simulink library "Arithmetic_Operations_Lib"  (R2023a)
settings: Solver=ode45  StartTime=0.0  StopTime=10.0  RelTol=1e-3  EnableMultiTasking=on
libraries: Miscellaneous x202
(part 3 of 4)

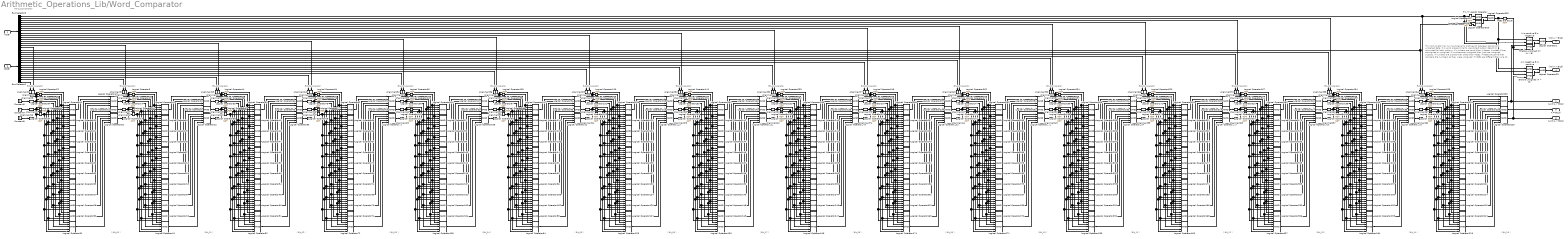
== system Arithmetic_Operations_Lib/Word_Comparator ==
  note: This comparator has no input signal to distinguish between signed and unsigned data. It is up to programmer to use correct output. Result is computed for both options.
      | If numbers are equal then it doesn`t matter if they are signed or unsigned.
      | If numbers are unsigned then just use unsigned outputs.
      | If numbers are signed then check their MSBs.
      | If MSBs are same then compare the numbers as they were unsigned.
      | If MSBs are different then one of the numbers is positive and the other one is negative. So we can immediatelly say which one is greater.
  note: Bit_Comparator
  note: ( Bit_00 )
  note: ( Bit_01 )
  note: Bit_Comparator
  note: ( Bit_02 )
  note: Bit_Comparator
  note: ( Bit_03 )
  note: Bit_Comparator
  note: ( Bit_06 )
  note: Bit_Comparator
  note: ( Bit_05 )
  note: ( Bit_04 )
  note: Bit_Comparator
  note: Bit_Comparator
  note: Bit_Comparator
  note: ( Bit_07 )
  note: Bit_Comparator
  note: Bit_Comparator
  note: ( Bit_09 )
  note: Bit_Comparator
  note: Bit_Comparator
  note: ( Bit_12 )
  note: ( Bit_13 )
  note: Bit_Comparator
  note: ( Bit_10 )
  note: ( Bit_14 )
  note: ( Bit_08 )
  note: Bit_Comparator
  note: Bit_Comparator
  note: ( Bit_11 )
  note: ( Bit_15 )
  note: Bit_Comparator
  note: Bit_Xor
  note: Word_Comparator
  A(2B) : Inport
  B(2B) : Inport  Port=2
  "A is negative B is positive " : Logic  Operator=NAND  IconShape=distinctive  AllPortsSameDT=off  OutDataTypeStr=boolean
  A is positive B is negative : Logic  Operator=NAND  IconShape=distinctive  AllPortsSameDT=off  OutDataTypeStr=boolean
  Alignment{1..75,77..81} (80 alike) : Miscellaneous/Alignment  SystemSampleTime=-1  VariantActivationTime=update diagram  Latency=0  AutoFrameSizeCalculation=off
  Bus Selector2 : BusSelector  OutputSignals=b15,b14,b13,b12,b11,b10,b09,b08,b07,b06,b05,b04,b03,b02,b01,b00
  Bus Selector3 : BusSelector  OutputSignals=b15,b14,b13,b12,b11,b10,b09,b08,b07,b06,b05,b04,b03,b02,b01,b00
  Constant3 : Constant  Value=0  OutDataTypeStr=int16
  Constant4 : Constant  OutDataTypeStr=int16
  Constant5 : Constant  Value=0  OutDataTypeStr=int16
  Enable unsigned (A < B) : Logic  Operator=NAND  IconShape=distinctive  AllPortsSameDT=off  OutDataTypeStr=boolean
  Enable unsigned (2) (A > B) : Logic  Operator=NAND  IconShape=distinctive  AllPortsSameDT=off  OutDataTypeStr=boolean
  Logical Operator{,1..2,21,29,43,63,93,95,118,140,183,208,236,238,261,283,303,317,319,326} (21 alike) : Logic  Operator=NAND  IconShape=distinctive  AllPortsSameDT=off  OutDataTypeStr=boolean
  Logical Operator{4..13,18..20,23..28,30..33,38..42,45..54,59..62,65..74,79..86,91..92,94,97..102,104..107,112..117,120..130,135..139,142..152,157..166,168..171,174,177..182,185..197,202..206,210..217,219..221,226..228,230..232,234..235,237,240..245,247..250,255..260,263..273,278..282,285..295,300..302,304..309,313,315..316,318,321,323..324} (224 alike) : Logic  Operator=NAND  Inputs=5  IconShape=distinctive  AllPortsSameDT=off  OutDataTypeStr=boolean
  Logical Operator{3,14..17,22,34..37,44,55..58,64,75..78,87..90,96,103,108..111,119,131..134,141,153..156,167,172..173,175..176,184,198..201,207,209,218,222..225,229,233,239,246,251..254,262,274..277,284,296..299,310..312,314,320,325,327} (82 alike) : Logic  Operator=NOT  IconShape=distinctive  AllPortsSameDT=off  OutDataTypeStr=boolean
  MSBs are equal : Logic  Operator=NOT  IconShape=distinctive  AllPortsSameDT=off  OutDataTypeStr=boolean
  (uint) A > B(1b) : Outport
  (uint) A < B(1b) : Outport  Port=2
  (int) A > B(1b) : Outport  Port=3
  (int) A < B(1b) : Outport  Port=4
  A = B(1b) : Outport  Port=5
  wires:
  Bus Selector3/15 -> Alignment3/1  "<b01>"
  A(2B)/1 -> Bus Selector3/1
  Bus Selector2/15 -> Alignment5/1  "<b01>"
  B(2B)/1 -> Bus Selector2/1
  "A is negative B is positive "/1 -> Logical Operator29/1
  A is positive B is negative/1 -> Logical Operator1/1
  Logical Operator29/1 -> (int) A < B(1b)/1
  Logical Operator1/1 -> (int) A > B(1b)/1
  Enable unsigned (A < B)/1 -> Logical Operator29/2
  Enable unsigned (2) (A > B)/1 -> Logical Operator1/2
  MSBs are equal/1 -> Enable unsigned (A < B)/1, Enable unsigned (2) (A > B)/2
  Logical Operator326/1 -> MSBs are equal/1, A is positive B is negative/1, "A is negative B is positive "/1
  Constant5/1 -> Alignment10/1
  Constant3/1 -> Alignment8/1
  Constant4/1 -> Alignment9/1
  Logical Operator30/1 -> Logical Operator32/4
  Logical Operator31/1 -> Logical Operator32/5
  Logical Operator33/1 -> Logical Operator32/1
  Logical Operator28/1 -> Logical Operator32/3
  Logical Operator27/1 -> Logical Operator32/2
  Logical Operator36/1 -> Logical Operator41/4, Logical Operator30/4, Logical Operator31/4, Logical Operator27/4, Logical Operator33/4, Logical Operator26/4, Logical Operator25/4, Logical Operator23/4
  Logical Operator37/1 -> Logical Operator41/5, Logical Operator28/5, Logical Operator30/5, Logical Operator39/5, Logical Operator38/5, Logical Operator26/5, Logical Operator25/5, Logical Operator24/5
  Logical Operator34/1 -> Logical Operator41/2, Logical Operator39/2, Logical Operator33/2, Logical Operator25/2, Logical Operator24/2, Logical Operator23/2
  Logical Operator22/1 -> Logical Operator41/1, Logical Operator30/1, Logical Operator28/1, Logical Operator27/1, Logical Operator33/1, Logical Operator39/1
  Logical Operator35/1 -> Logical Operator28/3, Logical Operator31/3, Logical Operator27/3, Logical Operator33/3, Logical Operator39/3, Logical Operator38/3, Logical Operator24/3, Logical Operator23/3
  Logical Operator38/1 -> Logical Operator21/1
  Logical Operator39/1 -> Logical Operator21/2
  Logical Operator26/1 -> Logical Operator40/5
  Logical Operator24/1 -> Logical Operator40/3
  Logical Operator23/1 -> Logical Operator40/2
  Logical Operator25/1 -> Logical Operator40/4
  Logical Operator41/1 -> Logical Operator40/1
  Alignment1/1 -> Logical Operator31/1, Logical Operator38/1, Logical Operator26/1, Logical Operator25/1, Logical Operator24/1, Logical Operator23/1, Logical Operator22/1
  Alignment2/1 -> Logical Operator30/2, Logical Operator31/2, Logical Operator28/2, Logical Operator27/2, Logical Operator38/2, Logical Operator26/2, Logical Operator34/1
  Alignment8/1 -> Logical Operator41/3, Logical Operator26/3, Logical Operator30/3, Logical Operator25/3, Logical Operator35/1
  Alignment9/1 -> Logical Operator36/1, Logical Operator28/4, Logical Operator39/4, Logical Operator38/4, Logical Operator24/4
  Alignment10/1 -> Logical Operator37/1, Logical Operator27/5, Logical Operator31/5, Logical Operator33/5, Logical Operator23/5
  Logical Operator42/1 -> Logical Operator20/1
  Logical Operator6/1 -> Logical Operator20/4
  Alignment3/1 -> Logical Operator11/1, Logical Operator18/1, Logical Operator7/1, Logical Operator6/1, Logical Operator5/1, Logical Operator4/1, Logical Operator3/1
  Logical Operator14/1 -> Logical Operator42/2, Logical Operator19/2, Logical Operator13/2, Logical Operator6/2, Logical Operator5/2, Logical Operator4/2
  Logical Operator3/1 -> Logical Operator42/1, Logical Operator10/1, Logical Operator9/1, Logical Operator8/1, Logical Operator13/1, Logical Operator19/1
  Logical Operator17/1 -> Logical Operator42/5, Logical Operator9/5, Logical Operator10/5, Logical Operator19/5, Logical Operator18/5, Logical Operator7/5, Logical Operator6/5, Logical Operator5/5
  Logical Operator15/1 -> Logical Operator9/3, Logical Operator11/3, Logical Operator8/3, Logical Operator13/3, Logical Operator19/3, Logical Operator18/3, Logical Operator5/3, Logical Operator4/3
  Logical Operator16/1 -> Logical Operator42/4, Logical Operator10/4, Logical Operator11/4, Logical Operator8/4, Logical Operator13/4, Logical Operator7/4, Logical Operator6/4, Logical Operator4/4
  Logical Operator9/1 -> Logical Operator12/3
  Logical Operator10/1 -> Logical Operator12/4
  Logical Operator18/1 -> Logical Operator2/1
  Logical Operator7/1 -> Logical Operator20/5
  Logical Operator13/1 -> Logical Operator12/1
  Alignment7/1 -> Logical Operator16/1, Logical Operator9/4, Logical Operator19/4, Logical Operator18/4, Logical Operator5/4
  Logical Operator11/1 -> Logical Operator12/5
  Alignment4/1 -> Logical Operator17/1, Logical Operator8/5, Logical Operator11/5, Logical Operator13/5, Logical Operator4/5
  Alignment5/1 -> Logical Operator10/2, Logical Operator11/2, Logical Operator9/2, Logical Operator8/2, Logical Operator18/2, Logical Operator7/2, Logical Operator14/1
  Logical Operator19/1 -> Logical Operator2/2
  Alignment6/1 -> Logical Operator42/3, Logical Operator7/3, Logical Operator10/3, Logical Operator6/3, Logical Operator15/1
  Logical Operator8/1 -> Logical Operator12/2
  Logical Operator5/1 -> Logical Operator20/3
  Logical Operator4/1 -> Logical Operator20/2
  Logical Operator62/1 -> Logical Operator61/1
  Logical Operator47/1 -> Logical Operator61/4
  Alignment11/1 -> Logical Operator52/1, Logical Operator59/1, Logical Operator48/1, Logical Operator47/1, Logical Operator46/1, Logical Operator45/1, Logical Operator44/1
  Logical Operator55/1 -> Logical Operator62/2, Logical Operator60/2, Logical Operator54/2, Logical Operator47/2, Logical Operator46/2, Logical Operator45/2
  Logical Operator44/1 -> Logical Operator62/1, Logical Operator51/1, Logical Operator50/1, Logical Operator49/1, Logical Operator54/1, Logical Operator60/1
  Logical Operator58/1 -> Logical Operator62/5, Logical Operator50/5, Logical Operator51/5, Logical Operator60/5, Logical Operator59/5, Logical Operator48/5, Logical Operator47/5, Logical Operator46/5
  Logical Operator56/1 -> Logical Operator50/3, Logical Operator52/3, Logical Operator49/3, Logical Operator54/3, Logical Operator60/3, Logical Operator59/3, Logical Operator46/3, Logical Operator45/3
  Logical Operator57/1 -> Logical Operator62/4, Logical Operator51/4, Logical Operator52/4, Logical Operator49/4, Logical Operator54/4, Logical Operator48/4, Logical Operator47/4, Logical Operator45/4
  Logical Operator50/1 -> Logical Operator53/3
  Logical Operator51/1 -> Logical Operator53/4
  Logical Operator59/1 -> Logical Operator43/1
  Logical Operator48/1 -> Logical Operator61/5
  Logical Operator54/1 -> Logical Operator53/1
  Alignment15/1 -> Logical Operator57/1, Logical Operator50/4, Logical Operator60/4, Logical Operator59/4, Logical Operator46/4
  Logical Operator52/1 -> Logical Operator53/5
  Alignment12/1 -> Logical Operator58/1, Logical Operator49/5, Logical Operator52/5, Logical Operator54/5, Logical Operator45/5
  Alignment13/1 -> Logical Operator51/2, Logical Operator52/2, Logical Operator50/2, Logical Operator49/2, Logical Operator59/2, Logical Operator48/2, Logical Operator55/1
  Logical Operator60/1 -> Logical Operator43/2
  Alignment14/1 -> Logical Operator62/3, Logical Operator48/3, Logical Operator51/3, Logical Operator47/3, Logical Operator56/1
  Logical Operator49/1 -> Logical Operator53/2
  Logical Operator46/1 -> Logical Operator61/3
  Logical Operator45/1 -> Logical Operator61/2
  Logical Operator82/1 -> Logical Operator81/1
  Logical Operator67/1 -> Logical Operator81/4
  Alignment16/1 -> Logical Operator72/1, Logical Operator79/1, Logical Operator68/1, Logical Operator67/1, Logical Operator66/1, Logical Operator65/1, Logical Operator64/1
  Logical Operator75/1 -> Logical Operator82/2, Logical Operator80/2, Logical Operator74/2, Logical Operator67/2, Logical Operator66/2, Logical Operator65/2
  Logical Operator64/1 -> Logical Operator82/1, Logical Operator71/1, Logical Operator70/1, Logical Operator69/1, Logical Operator74/1, Logical Operator80/1
  Logical Operator78/1 -> Logical Operator82/5, Logical Operator70/5, Logical Operator71/5, Logical Operator80/5, Logical Operator79/5, Logical Operator68/5, Logical Operator67/5, Logical Operator66/5
  Logical Operator76/1 -> Logical Operator70/3, Logical Operator72/3, Logical Operator69/3, Logical Operator74/3, Logical Operator80/3, Logical Operator79/3, Logical Operator66/3, Logical Operator65/3
  Logical Operator77/1 -> Logical Operator82/4, Logical Operator71/4, Logical Operator72/4, Logical Operator69/4, Logical Operator74/4, Logical Operator68/4, Logical Operator67/4, Logical Operator65/4
  Logical Operator70/1 -> Logical Operator73/3
  Logical Operator71/1 -> Logical Operator73/4
  Logical Operator79/1 -> Logical Operator63/1
  Logical Operator68/1 -> Logical Operator81/5
  Logical Operator74/1 -> Logical Operator73/1
  Alignment20/1 -> Logical Operator77/1, Logical Operator70/4, Logical Operator80/4, Logical Operator79/4, Logical Operator66/4
  Logical Operator72/1 -> Logical Operator73/5
  Alignment17/1 -> Logical Operator78/1, Logical Operator69/5, Logical Operator72/5, Logical Operator74/5, Logical Operator65/5
  Alignment18/1 -> Logical Operator71/2, Logical Operator72/2, Logical Operator70/2, Logical Operator69/2, Logical Operator79/2, Logical Operator68/2, Logical Operator75/1
  Logical Operator80/1 -> Logical Operator63/2
  Alignment19/1 -> Logical Operator82/3, Logical Operator68/3, Logical Operator71/3, Logical Operator67/3, Logical Operator76/1
  Logical Operator69/1 -> Logical Operator73/2
  Logical Operator66/1 -> Logical Operator81/3
  Logical Operator65/1 -> Logical Operator81/2
  Logical Operator61/1 -> Alignment19/1
  Logical Operator43/1 -> Alignment20/1
  Logical Operator53/1 -> Alignment17/1
  Logical Operator20/1 -> Alignment14/1
  Logical Operator2/1 -> Alignment15/1
  Logical Operator12/1 -> Alignment12/1
  Logical Operator40/1 -> Alignment6/1
  Logical Operator21/1 -> Alignment7/1
  Logical Operator32/1 -> Alignment4/1
  Logical Operator145/1 -> Logical Operator160/5
  Logical Operator157/1 -> Logical Operator140/1
  Logical Operator152/1 -> Logical Operator151/1
  Logical Operator149/1 -> Logical Operator151/4
  Logical Operator154/1 -> Logical Operator148/3, Logical Operator150/3, Logical Operator146/3, Logical Operator152/3, Logical Operator159/3, Logical Operator157/3, Logical Operator143/3, Logical Operator142/3
  Logical Operator155/1 -> Logical Operator161/4, Logical Operator149/4, Logical Operator150/4, Logical Operator146/4, Logical Operator152/4, Logical Operator145/4, Logical Operator144/4, Logical Operator142/4
  Logical Operator148/1 -> Logical Operator151/3
  Alignment28/1 -> Logical Operator150/1, Logical Operator157/1, Logical Operator145/1, Logical Operator144/1, Logical Operator143/1, Logical Operator142/1, Logical Operator141/1
  Logical Operator144/1 -> Logical Operator160/4
  Logical Operator118/1 -> Alignment33/1
  Logical Operator106/1 -> Alignment35/1
  Logical Operator117/1 -> Logical Operator94/1
  Logical Operator161/1 -> Logical Operator160/1
  Logical Operator129/1 -> Alignment29/1
  Logical Operator124/1 -> Logical Operator129/2
  Alignment26/1 -> Logical Operator139/3, Logical Operator123/3, Logical Operator127/3, Logical Operator122/3, Logical Operator132/1
  Alignment25/1 -> Logical Operator127/2, Logical Operator128/2, Logical Operator126/2, Logical Operator124/2, Logical Operator135/2, Logical Operator123/2, Logical Operator131/1
  Logical Operator137/1 -> Logical Operator118/2
  Alignment27/1 -> Logical Operator133/1, Logical Operator126/4, Logical Operator137/4, Logical Operator135/4, Logical Operator121/4
  Alignment24/1 -> Logical Operator134/1, Logical Operator124/5, Logical Operator128/5, Logical Operator130/5, Logical Operator120/5
  Logical Operator128/1 -> Logical Operator129/5
  Alignment33/1 -> Logical Operator155/1, Logical Operator148/4, Logical Operator159/4, Logical Operator157/4, Logical Operator143/4
  Logical Operator130/1 -> Logical Operator129/1
  Logical Operator141/1 -> Logical Operator161/1, Logical Operator149/1, Logical Operator148/1, Logical Operator146/1, Logical Operator152/1, Logical Operator159/1
  Logical Operator119/1 -> Logical Operator139/1, Logical Operator127/1, Logical Operator126/1, Logical Operator124/1, Logical Operator130/1, Logical Operator137/1
  Alignment23/1 -> Logical Operator128/1, Logical Operator135/1, Logical Operator123/1, Logical Operator122/1, Logical Operator121/1, Logical Operator120/1, Logical Operator119/1
  Logical Operator131/1 -> Logical Operator139/2, Logical Operator137/2, Logical Operator130/2, Logical Operator122/2, Logical Operator121/2, Logical Operator120/2
  Alignment29/1 -> Logical Operator156/1, Logical Operator146/5, Logical Operator150/5, Logical Operator152/5, Logical Operator142/5
  Logical Operator156/1 -> Logical Operator161/5, Logical Operator148/5, Logical Operator149/5, Logical Operator159/5, Logical Operator157/5, Logical Operator145/5, Logical Operator144/5, Logical Operator143/5
  Logical Operator138/1 -> Alignment31/1
  Logical Operator123/1 -> Logical Operator138/5
  Alignment36/1 -> Logical Operator83/2, Logical Operator84/2, Logical Operator162/2, Logical Operator158/2, Logical Operator91/2, Logical Operator147/2, Logical Operator87/1
  Logical Operator93/1 -> Alignment27/1
  Alignment35/1 -> Logical Operator90/1, Logical Operator158/5, Logical Operator84/5, Logical Operator86/5, Logical Operator114/5
  Alignment38/1 -> Logical Operator89/1, Logical Operator162/4, Logical Operator92/4, Logical Operator91/4, Logical Operator125/4
  Logical Operator95/1 -> Alignment38/1
  Logical Operator94/1 -> Alignment26/1
  Logical Operator99/1 -> Logical Operator115/4
  Logical Operator121/1 -> Logical Operator138/3
  Alignment21/1 -> Logical Operator105/1, Logical Operator112/1, Logical Operator100/1, Logical Operator99/1, Logical Operator98/1, Logical Operator97/1, Logical Operator96/1
  Logical Operator136/1 -> Logical Operator94/4
  Logical Operator108/1 -> Logical Operator116/2, Logical Operator113/2, Logical Operator107/2, Logical Operator99/2, Logical Operator98/2, Logical Operator97/2
  Logical Operator84/1 -> Logical Operator85/5
  Logical Operator96/1 -> Logical Operator116/1, Logical Operator104/1, Logical Operator102/1, Logical Operator101/1, Logical Operator107/1, Logical Operator113/1
  Logical Operator111/1 -> Logical Operator116/5, Logical Operator102/5, Logical Operator104/5, Logical Operator113/5, Logical Operator112/5, Logical Operator100/5, Logical Operator99/5, Logical Operator98/5
  Logical Operator126/1 -> Logical Operator129/3
  Logical Operator110/1 -> Logical Operator116/4, Logical Operator104/4, Logical Operator105/4, Logical Operator101/4, Logical Operator107/4, Logical Operator100/4, Logical Operator99/4, Logical Operator97/4
  Logical Operator107/1 -> Logical Operator106/1
  Logical Operator102/1 -> Logical Operator106/3
  Logical Operator105/1 -> Logical Operator106/5
  Logical Operator113/1 -> Logical Operator95/2
  Logical Operator100/1 -> Logical Operator115/5
  Logical Operator142/1 -> Logical Operator160/2
  Logical Operator135/1 -> Logical Operator118/1
  Logical Operator127/1 -> Logical Operator129/4
  Logical Operator109/1 -> Logical Operator102/3, Logical Operator105/3, Logical Operator101/3, Logical Operator107/3, Logical Operator113/3, Logical Operator112/3, Logical Operator98/3, Logical Operator97/3
  Logical Operator133/1 -> Logical Operator139/4, Logical Operator127/4, Logical Operator128/4, Logical Operator124/4, Logical Operator130/4, Logical Operator123/4, Logical Operator122/4, Logical Operator120/4
  Logical Operator92/1 -> Logical Operator93/2
  Logical Operator116/1 -> Logical Operator115/1
  Logical Operator90/1 -> Logical Operator117/5, Logical Operator162/5, Logical Operator83/5, Logical Operator92/5, Logical Operator91/5, Logical Operator147/5, Logical Operator136/5, Logical Operator125/5
  Logical Operator85/1 -> Alignment24/1
  Logical Operator104/1 -> Logical Operator106/4
  Logical Operator132/1 -> Logical Operator126/3, Logical Operator128/3, Logical Operator124/3, Logical Operator130/3, Logical Operator137/3, Logical Operator135/3, Logical Operator121/3, Logical Operator120/3
  Logical Operator115/1 -> Alignment37/1
  Logical Operator146/1 -> Logical Operator151/2
  Alignment31/1 -> Logical Operator161/3, Logical Operator145/3, Logical Operator149/3, Logical Operator144/3, Logical Operator154/1
  Logical Operator150/1 -> Logical Operator151/5
  Logical Operator112/1 -> Logical Operator95/1
  Logical Operator139/1 -> Logical Operator138/1
  Alignment30/1 -> Logical Operator149/2, Logical Operator150/2, Logical Operator148/2, Logical Operator146/2, Logical Operator157/2, Logical Operator145/2, Logical Operator153/1
  Logical Operator158/1 -> Logical Operator85/2
  Logical Operator86/1 -> Logical Operator85/1
  Logical Operator147/1 -> Logical Operator94/5
  Logical Operator162/1 -> Logical Operator85/3
  Logical Operator87/1 -> Logical Operator117/2, Logical Operator92/2, Logical Operator86/2, Logical Operator136/2, Logical Operator125/2, Logical Operator114/2
  Logical Operator114/1 -> Logical Operator94/2
  Logical Operator83/1 -> Logical Operator85/4
  Logical Operator91/1 -> Logical Operator93/1
  Alignment37/1 -> Logical Operator117/3, Logical Operator147/3, Logical Operator83/3, Logical Operator136/3, Logical Operator88/1
  Logical Operator159/1 -> Logical Operator140/2
  Logical Operator143/1 -> Logical Operator160/3
  Logical Operator88/1 -> Logical Operator162/3, Logical Operator84/3, Logical Operator158/3, Logical Operator86/3, Logical Operator92/3, Logical Operator91/3, Logical Operator125/3, Logical Operator114/3
  Alignment34/1 -> Logical Operator84/1, Logical Operator91/1, Logical Operator147/1, Logical Operator136/1, Logical Operator125/1, Logical Operator114/1, Logical Operator103/1
  Alignment40/1 -> Logical Operator110/1, Logical Operator102/4, Logical Operator113/4, Logical Operator112/4, Logical Operator98/4
  Alignment22/1 -> Logical Operator111/1, Logical Operator101/5, Logical Operator105/5, Logical Operator107/5, Logical Operator97/5
  Logical Operator89/1 -> Logical Operator117/4, Logical Operator83/4, Logical Operator84/4, Logical Operator158/4, Logical Operator86/4, Logical Operator147/4, Logical Operator136/4, Logical Operator114/4
  Logical Operator120/1 -> Logical Operator138/2
  Alignment32/1 -> Logical Operator104/2, Logical Operator105/2, Logical Operator102/2, Logical Operator101/2, Logical Operator112/2, Logical Operator100/2, Logical Operator108/1
  Logical Operator103/1 -> Logical Operator117/1, Logical Operator83/1, Logical Operator162/1, Logical Operator158/1, Logical Operator86/1, Logical Operator92/1
  Logical Operator153/1 -> Logical Operator161/2, Logical Operator159/2, Logical Operator152/2, Logical Operator144/2, Logical Operator143/2, Logical Operator142/2
  Alignment39/1 -> Logical Operator116/3, Logical Operator100/3, Logical Operator104/3, Logical Operator99/3, Logical Operator109/1
  Logical Operator101/1 -> Logical Operator106/2
  Logical Operator134/1 -> Logical Operator139/5, Logical Operator126/5, Logical Operator127/5, Logical Operator137/5, Logical Operator135/5, Logical Operator123/5, Logical Operator122/5, Logical Operator121/5
  Logical Operator98/1 -> Logical Operator115/3
  Logical Operator97/1 -> Logical Operator115/2
  Logical Operator122/1 -> Logical Operator138/4
  Logical Operator125/1 -> Logical Operator94/3
  Logical Operator288/1 -> Logical Operator304/5
  Logical Operator300/1 -> Logical Operator283/1
  Logical Operator295/1 -> Logical Operator294/1
  Logical Operator292/1 -> Logical Operator294/4
  Logical Operator297/1 -> Logical Operator291/3, Logical Operator293/3, Logical Operator289/3, Logical Operator295/3, Logical Operator302/3, Logical Operator300/3, Logical Operator286/3, Logical Operator285/3
  Logical Operator298/1 -> Logical Operator305/4, Logical Operator292/4, Logical Operator293/4, Logical Operator289/4, Logical Operator295/4, Logical Operator288/4, Logical Operator287/4, Logical Operator285/4
  Logical Operator291/1 -> Logical Operator294/3
  Alignment53/1 -> Logical Operator298/1, Logical Operator291/4, Logical Operator302/4, Logical Operator300/4, Logical Operator286/4
  Logical Operator299/1 -> Logical Operator305/5, Logical Operator291/5, Logical Operator292/5, Logical Operator302/5, Logical Operator300/5, Logical Operator288/5, Logical Operator287/5, Logical Operator286/5
  Logical Operator287/1 -> Logical Operator304/4
  Logical Operator305/1 -> Logical Operator304/1
  Logical Operator236/1 -> Alignment47/1
  Logical Operator238/1 -> Alignment79/1
  Logical Operator249/1 -> Alignment74/1
  Logical Operator272/1 -> Alignment49/1
  Logical Operator264/1 -> Logical Operator281/3
  Logical Operator267/1 -> Logical Operator272/2
  Alignment46/1 -> Logical Operator282/3, Logical Operator266/3, Logical Operator270/3, Logical Operator265/3, Logical Operator275/1
  Alignment45/1 -> Logical Operator270/2, Logical Operator271/2, Logical Operator269/2, Logical Operator267/2, Logical Operator278/2, Logical Operator266/2, Logical Operator274/1
  Alignment47/1 -> Logical Operator276/1, Logical Operator269/4, Logical Operator280/4, Logical Operator278/4, Logical Operator264/4
  Logical Operator271/1 -> Logical Operator272/5
  Logical Operator266/1 -> Logical Operator281/5
  Logical Operator296/1 -> Logical Operator305/2, Logical Operator302/2, Logical Operator295/2, Logical Operator287/2, Logical Operator286/2, Logical Operator285/2
  Logical Operator277/1 -> Logical Operator282/5, Logical Operator269/5, Logical Operator270/5, Logical Operator280/5, Logical Operator278/5, Logical Operator266/5, Logical Operator265/5, Logical Operator264/5
  Logical Operator262/1 -> Logical Operator282/1, Logical Operator270/1, Logical Operator269/1, Logical Operator267/1, Logical Operator273/1, Logical Operator280/1
  Alignment43/1 -> Logical Operator271/1, Logical Operator278/1, Logical Operator266/1, Logical Operator265/1, Logical Operator264/1, Logical Operator263/1, Logical Operator262/1
  Alignment49/1 -> Logical Operator299/1, Logical Operator289/5, Logical Operator293/5, Logical Operator295/5, Logical Operator285/5
  Logical Operator281/1 -> Alignment51/1
  Logical Operator197/1 -> Logical Operator195/1
  Alignment57/1 -> Logical Operator201/1, Logical Operator190/5, Logical Operator194/5, Logical Operator197/5, Logical Operator186/5
  Logical Operator189/1 -> Logical Operator205/5
  Logical Operator194/1 -> Logical Operator195/5
  Logical Operator204/1 -> Logical Operator183/2
  Alignment58/1 -> Logical Operator193/2, Logical Operator194/2, Logical Operator192/2, Logical Operator190/2, Logical Operator202/2, Logical Operator189/2, Logical Operator198/1
  Logical Operator190/1 -> Logical Operator195/2
  Logical Operator170/1 -> Alignment69/1
  Logical Operator182/1 -> Logical Operator318/1
  Logical Operator284/1 -> Logical Operator305/1, Logical Operator292/1, Logical Operator291/1, Logical Operator289/1, Logical Operator295/1, Logical Operator302/1
  Logical Operator260/1 -> Logical Operator237/1
  Logical Operator184/1 -> Logical Operator206/1, Logical Operator193/1, Logical Operator192/1, Logical Operator190/1, Logical Operator197/1, Logical Operator204/1
  Logical Operator166/1 -> Logical Operator170/3
  Logical Operator175/1 -> Logical Operator181/4, Logical Operator168/4, Logical Operator169/4, Logical Operator165/4, Logical Operator171/4, Logical Operator164/4, Logical Operator324/4, Logical Operator321/4
  Logical Operator192/1 -> Logical Operator195/3
  Alignment44/1 -> Logical Operator277/1, Logical Operator267/5, Logical Operator271/5, Logical Operator273/5, Logical Operator263/5
  Logical Operator307/1 -> Logical Operator308/5
  Alignment48/1 -> Logical Operator293/1, Logical Operator300/1, Logical Operator288/1, Logical Operator287/1, Logical Operator286/1, Logical Operator285/1, Logical Operator284/1
  Logical Operator172/1 -> Logical Operator181/2, Logical Operator178/2, Logical Operator171/2, Logical Operator324/2, Logical Operator323/2, Logical Operator321/2
  Logical Operator203/1 -> Logical Operator318/4
  Alignment54/1 -> Logical Operator169/1, Logical Operator177/1, Logical Operator164/1, Logical Operator324/1, Logical Operator323/1, Logical Operator321/1, Logical Operator320/1
  Logical Operator169/1 -> Logical Operator170/5
  Logical Operator178/1 -> Logical Operator319/2
  Logical Operator200/1 -> Logical Operator206/4, Logical Operator193/4, Logical Operator194/4, Logical Operator190/4, Logical Operator197/4, Logical Operator189/4, Logical Operator188/4, Logical Operator186/4
  Logical Operator186/1 -> Logical Operator205/2
  Logical Operator312/1 -> Logical Operator182/4, Logical Operator306/4, Logical Operator307/4, Logical Operator227/4, Logical Operator309/4, Logical Operator215/4, Logical Operator203/4, Logical Operator179/4
  Alignment75/1 -> Logical Operator175/1, Logical Operator166/4, Logical Operator178/4, Logical Operator177/4, Logical Operator323/4
  Logical Operator273/1 -> Logical Operator272/1
  Alignment55/1 -> Logical Operator176/1, Logical Operator165/5, Logical Operator169/5, Logical Operator171/5, Logical Operator321/5
  Alignment68/1 -> Logical Operator307/1, Logical Operator315/1, Logical Operator215/1, Logical Operator203/1, Logical Operator191/1, Logical Operator179/1, Logical Operator167/1
  Logical Operator280/1 -> Logical Operator261/2
  Logical Operator232/1 -> Logical Operator308/3
  Logical Operator193/1 -> Logical Operator195/4
  Logical Operator177/1 -> Logical Operator319/1
  Logical Operator215/1 -> Logical Operator318/5
  Logical Operator199/1 -> Logical Operator192/3, Logical Operator194/3, Logical Operator190/3, Logical Operator197/3, Logical Operator204/3, Logical Operator202/3, Logical Operator187/3, Logical Operator186/3
  Logical Operator310/1 -> Logical Operator182/2, Logical Operator316/2, Logical Operator309/2, Logical Operator203/2, Logical Operator191/2, Logical Operator179/2
  Logical Operator314/1 -> Logical Operator182/5, Logical Operator232/5, Logical Operator306/5, Logical Operator316/5, Logical Operator315/5, Logical Operator215/5, Logical Operator203/5, Logical Operator191/5
  Logical Operator308/1 -> Alignment57/1
  Logical Operator181/1 -> Logical Operator180/1
  Logical Operator165/1 -> Logical Operator170/2
  Logical Operator315/1 -> Logical Operator317/1
  Logical Operator311/1 -> Logical Operator232/3, Logical Operator307/3, Logical Operator227/3, Logical Operator309/3, Logical Operator316/3, Logical Operator315/3, Logical Operator191/3, Logical Operator179/3
  Logical Operator164/1 -> Logical Operator180/5
  Alignment74/1 -> Logical Operator233/1, Logical Operator301/5, Logical Operator174/5, Logical Operator196/5, Logical Operator257/5
  Alignment79/1 -> Logical Operator229/1, Logical Operator313/4, Logical Operator235/4, Logical Operator234/4, Logical Operator268/4
  Logical Operator316/1 -> Logical Operator317/2
  Logical Operator167/1 -> Logical Operator182/1, Logical Operator306/1, Logical Operator232/1, Logical Operator227/1, Logical Operator309/1, Logical Operator316/1
  Logical Operator274/1 -> Logical Operator282/2, Logical Operator280/2, Logical Operator273/2, Logical Operator265/2, Logical Operator264/2, Logical Operator263/2
  Logical Operator198/1 -> Logical Operator206/2, Logical Operator204/2, Logical Operator197/2, Logical Operator188/2, Logical Operator187/2, Logical Operator186/2
  Logical Operator237/1 -> Alignment46/1
  Logical Operator242/1 -> Logical Operator258/4
  Alignment41/1 -> Logical Operator248/1, Logical Operator255/1, Logical Operator243/1, Logical Operator242/1, Logical Operator241/1, Logical Operator240/1, Logical Operator239/1
  Alignment60/1 -> Logical Operator200/1, Logical Operator192/4, Logical Operator204/4, Logical Operator202/4, Logical Operator187/4
  Logical Operator251/1 -> Logical Operator259/2, Logical Operator256/2, Logical Operator250/2, Logical Operator242/2, Logical Operator241/2, Logical Operator240/2
  Logical Operator168/1 -> Logical Operator170/4
  Logical Operator174/1 -> Logical Operator185/5
  Logical Operator239/1 -> Logical Operator259/1, Logical Operator247/1, Logical Operator245/1, Logical Operator244/1, Logical Operator250/1, Logical Operator256/1
  Logical Operator254/1 -> Logical Operator259/5, Logical Operator245/5, Logical Operator247/5, Logical Operator256/5, Logical Operator255/5, Logical Operator243/5, Logical Operator242/5, Logical Operator241/5
  Logical Operator261/1 -> Alignment53/1
  Alignment69/1 -> Logical Operator314/1, Logical Operator227/5, Logical Operator307/5, Logical Operator309/5, Logical Operator179/5
  Logical Operator320/1 -> Logical Operator181/1, Logical Operator168/1, Logical Operator166/1, Logical Operator165/1, Logical Operator171/1, Logical Operator178/1
  Logical Operator306/1 -> Logical Operator308/4
  Logical Operator269/1 -> Logical Operator272/3
  Alignment71/1 -> Logical Operator182/3, Logical Operator215/3, Logical Operator306/3, Logical Operator203/3, Logical Operator311/1
  Logical Operator250/1 -> Logical Operator249/1
  Logical Operator309/1 -> Logical Operator308/1
  Logical Operator245/1 -> Logical Operator249/3
  Logical Operator248/1 -> Logical Operator249/5
  Alignment73/1 -> Logical Operator181/3, Logical Operator164/3, Logical Operator168/3, Logical Operator324/3, Logical Operator173/1
  Logical Operator256/1 -> Logical Operator238/2
  Logical Operator243/1 -> Logical Operator258/5
  Logical Operator285/1 -> Logical Operator304/2
  Alignment56/1 -> Logical Operator194/1, Logical Operator202/1, Logical Operator189/1, Logical Operator188/1, Logical Operator187/1, Logical Operator186/1, Logical Operator184/1
  Logical Operator278/1 -> Logical Operator261/1
  Logical Operator270/1 -> Logical Operator272/4
  Logical Operator252/1 -> Logical Operator245/3, Logical Operator248/3, Logical Operator244/3, Logical Operator250/3, Logical Operator256/3, Logical Operator255/3, Logical Operator241/3, Logical Operator240/3
  Logical Operator235/1 -> Logical Operator236/2
  Logical Operator202/1 -> Logical Operator183/1
  Logical Operator259/1 -> Logical Operator258/1
  Logical Operator233/1 -> Logical Operator260/5, Logical Operator313/5, Logical Operator163/5, Logical Operator235/5, Logical Operator234/5, Logical Operator290/5, Logical Operator279/5, Logical Operator268/5
  Logical Operator185/1 -> Alignment44/1
  Logical Operator247/1 -> Logical Operator249/4
  Logical Operator275/1 -> Logical Operator269/3, Logical Operator271/3, Logical Operator267/3, Logical Operator273/3, Logical Operator280/3, Logical Operator278/3, Logical Operator264/3, Logical Operator263/3
  Logical Operator227/1 -> Logical Operator308/2
  Logical Operator318/1 -> Alignment59/1
  Logical Operator258/1 -> Alignment78/1
  Alignment51/1 -> Logical Operator305/3, Logical Operator288/3, Logical Operator292/3, Logical Operator287/3, Logical Operator297/1
  Logical Operator324/1 -> Logical Operator180/4
  Logical Operator179/1 -> Logical Operator318/2
  Logical Operator293/1 -> Logical Operator294/5
  Logical Operator282/1 -> Logical Operator281/1
  Alignment50/1 -> Logical Operator292/2, Logical Operator293/2, Logical Operator291/2, Logical Operator289/2, Logical Operator300/2, Logical Operator288/2, Logical Operator296/1
  Alignment78/1 -> Logical Operator260/3, Logical Operator290/3, Logical Operator163/3, Logical Operator279/3, Logical Operator218/1
  Logical Operator301/1 -> Logical Operator185/2
  Logical Operator171/1 -> Logical Operator170/1
  Logical Operator218/1 -> Logical Operator313/3, Logical Operator174/3, Logical Operator301/3, Logical Operator196/3, Logical Operator235/3, Logical Operator234/3, Logical Operator268/3, Logical Operator257/3
  Logical Operator286/1 -> Logical Operator304/3
  Logical Operator196/1 -> Logical Operator185/1
  Logical Operator290/1 -> Logical Operator237/5
  Logical Operator234/1 -> Logical Operator236/1
  Logical Operator163/1 -> Logical Operator185/4
  Logical Operator313/1 -> Logical Operator185/3
  Logical Operator207/1 -> Logical Operator260/2, Logical Operator235/2, Logical Operator196/2, Logical Operator279/2, Logical Operator268/2, Logical Operator257/2
  Logical Operator229/1 -> Logical Operator260/4, Logical Operator163/4, Logical Operator174/4, Logical Operator301/4, Logical Operator196/4, Logical Operator290/4, Logical Operator279/4, Logical Operator257/4
  Logical Operator206/1 -> Logical Operator205/1
  Logical Operator191/1 -> Logical Operator318/3
  Logical Operator188/1 -> Logical Operator205/4
  Logical Operator289/1 -> Logical Operator294/2
  Logical Operator201/1 -> Logical Operator206/5, Logical Operator192/5, Logical Operator193/5, Logical Operator204/5, Logical Operator202/5, Logical Operator189/5, Logical Operator188/5, Logical Operator187/5
  Alignment77/1 -> Logical Operator163/2, Logical Operator174/2, Logical Operator313/2, Logical Operator301/2, Logical Operator234/2, Logical Operator290/2, Logical Operator207/1
  Logical Operator321/1 -> Logical Operator180/2
  Logical Operator323/1 -> Logical Operator180/3
  Logical Operator319/1 -> Alignment72/1
  Alignment42/1 -> Logical Operator254/1, Logical Operator244/5, Logical Operator248/5, Logical Operator250/5, Logical Operator240/5
  Logical Operator302/1 -> Logical Operator283/2
  Alignment63/1 -> Logical Operator174/1, Logical Operator234/1, Logical Operator290/1, Logical Operator279/1, Logical Operator268/1, Logical Operator257/1, Logical Operator246/1
  Alignment81/1 -> Logical Operator253/1, Logical Operator245/4, Logical Operator256/4, Logical Operator255/4, Logical Operator241/4
  Alignment80/1 -> Logical Operator259/3, Logical Operator243/3, Logical Operator247/3, Logical Operator242/3, Logical Operator252/1
  Alignment66/1 -> Logical Operator168/2, Logical Operator169/2, Logical Operator166/2, Logical Operator165/2, Logical Operator177/2, Logical Operator164/2, Logical Operator172/1
  Logical Operator246/1 -> Logical Operator260/1, Logical Operator163/1, Logical Operator313/1, Logical Operator301/1, Logical Operator196/1, Logical Operator235/1
  Logical Operator276/1 -> Logical Operator282/4, Logical Operator270/4, Logical Operator271/4, Logical Operator267/4, Logical Operator273/4, Logical Operator266/4, Logical Operator265/4, Logical Operator263/4
  Logical Operator180/1 -> Alignment71/1
  Logical Operator244/1 -> Logical Operator249/2
  Logical Operator173/1 -> Logical Operator166/3, Logical Operator169/3, Logical Operator165/3, Logical Operator171/3, Logical Operator178/3, Logical Operator177/3, Logical Operator323/3, Logical Operator321/3
  Logical Operator255/1 -> Logical Operator238/1
  Alignment52/1 -> Logical Operator247/2, Logical Operator248/2, Logical Operator245/2, Logical Operator244/2, Logical Operator255/2, Logical Operator243/2, Logical Operator251/1
  Logical Operator263/1 -> Logical Operator281/2
  Logical Operator265/1 -> Logical Operator281/4
  Logical Operator268/1 -> Logical Operator237/3
  Logical Operator240/1 -> Logical Operator258/2
  Logical Operator241/1 -> Logical Operator258/3
  Logical Operator257/1 -> Logical Operator237/2
  Alignment72/1 -> Logical Operator312/1, Logical Operator232/4, Logical Operator316/4, Logical Operator315/4, Logical Operator191/4
  Logical Operator253/1 -> Logical Operator259/4, Logical Operator247/4, Logical Operator248/4, Logical Operator244/4, Logical Operator250/4, Logical Operator243/4, Logical Operator242/4, Logical Operator240/4
  Alignment59/1 -> Logical Operator206/3, Logical Operator189/3, Logical Operator193/3, Logical Operator188/3, Logical Operator199/1
  Logical Operator187/1 -> Logical Operator205/3
  Logical Operator279/1 -> Logical Operator237/4
  Logical Operator176/1 -> Logical Operator181/5, Logical Operator166/5, Logical Operator168/5, Logical Operator178/5, Logical Operator177/5, Logical Operator164/5, Logical Operator324/5, Logical Operator323/5
  Logical Operator317/1 -> Alignment60/1
  Alignment70/1 -> Logical Operator306/2, Logical Operator307/2, Logical Operator232/2, Logical Operator227/2, Logical Operator315/2, Logical Operator215/2, Logical Operator310/1
  Logical Operator81/1 -> Alignment39/1
  Logical Operator63/1 -> Alignment40/1
  Logical Operator73/1 -> Alignment22/1
  Logical Operator160/1 -> Alignment80/1
  Logical Operator140/1 -> Alignment81/1
  Logical Operator151/1 -> Alignment42/1
  Logical Operator304/1 -> Alignment73/1
  Logical Operator283/1 -> Alignment75/1
  Logical Operator294/1 -> Alignment55/1
  Bus Selector2/16 -> Alignment2/1  "<b00>"
  Bus Selector3/16 -> Alignment1/1  "<b00>"
  Bus Selector3/14 -> Alignment11/1  "<b02>"
  Bus Selector3/13 -> Alignment16/1  "<b03>"
  Bus Selector3/12 -> Alignment21/1  "<b04>"
  Bus Selector3/11 -> Alignment34/1  "<b05>"
  Bus Selector3/10 -> Alignment23/1  "<b06>"
  Bus Selector3/9 -> Alignment28/1  "<b07>"
  Bus Selector3/8 -> Alignment41/1  "<b08>"
  Bus Selector3/7 -> Alignment63/1  "<b09>"
  Bus Selector3/6 -> Alignment43/1  "<b10>"
  Bus Selector3/5 -> Alignment48/1  "<b11>"
  Bus Selector3/4 -> Alignment54/1  "<b12>"
  Bus Selector3/3 -> Alignment68/1  "<b13>"
  Bus Selector3/2 -> Alignment56/1  "<b14>"
  Bus Selector2/14 -> Alignment13/1  "<b02>"
  Bus Selector2/13 -> Alignment18/1  "<b03>"
  Bus Selector2/12 -> Alignment32/1  "<b04>"
  Bus Selector2/11 -> Alignment36/1  "<b05>"
  Bus Selector2/10 -> Alignment25/1  "<b06>"
  Bus Selector2/9 -> Alignment30/1  "<b07>"
  Bus Selector2/8 -> Alignment52/1  "<b08>"
  Bus Selector2/7 -> Alignment77/1  "<b09>"
  Bus Selector2/6 -> Alignment45/1  "<b10>"
  Bus Selector2/5 -> Alignment50/1  "<b11>"
  Bus Selector2/4 -> Alignment66/1  "<b12>"
  Bus Selector2/3 -> Alignment70/1  "<b13>"
  Bus Selector2/2 -> Alignment58/1  "<b14>"
  Bus Selector3/1 -> "A is negative B is positive "/2, Logical Operator303/1, Logical Operator327/1, Alignment61/1  "<b14>"
  Logical Operator183/1 -> Alignment67/1
  Logical Operator211/1 -> Logical Operator230/3
  Alignment65/1 -> Logical Operator231/3, Logical Operator213/3, Logical Operator217/3, Logical Operator212/3, Logical Operator223/1
  Logical Operator210/1 -> Logical Operator230/2
  Logical Operator224/1 -> Logical Operator231/4, Logical Operator217/4, Logical Operator219/4, Logical Operator214/4, Logical Operator221/4, Logical Operator213/4, Logical Operator212/4, Logical Operator210/4
  Logical Operator216/1 -> Logical Operator220/3
  Logical Operator209/1 -> Logical Operator231/1, Logical Operator217/1, Logical Operator216/1, Logical Operator214/1, Logical Operator221/1, Logical Operator228/1
  Alignment64/1 -> Logical Operator217/2, Logical Operator219/2, Logical Operator216/2, Logical Operator214/2, Logical Operator226/2, Logical Operator213/2, Logical Operator222/1
  Logical Operator219/1 -> Logical Operator220/5
  Logical Operator228/1 -> Logical Operator208/2
  Alignment62/1 -> Logical Operator225/1, Logical Operator214/5, Logical Operator219/5, Logical Operator221/5, Logical Operator210/5
  Logical Operator214/1 -> Logical Operator220/2
  Logical Operator213/1 -> Logical Operator230/5
  Logical Operator221/1 -> Logical Operator220/1
  Logical Operator195/1 -> Alignment62/1
  Logical Operator223/1 -> Logical Operator216/3, Logical Operator219/3, Logical Operator214/3, Logical Operator221/3, Logical Operator228/3, Logical Operator226/3, Logical Operator211/3, Logical Operator210/3
  Bus Selector2/1 -> Logical Operator325/1, A is positive B is negative/2, Logical Operator/2, Alignment64/1  "<b14>"
  Logical Operator212/1 -> Logical Operator230/4
  Logical Operator225/1 -> Logical Operator231/5, Logical Operator216/5, Logical Operator217/5, Logical Operator228/5, Logical Operator226/5, Logical Operator213/5, Logical Operator212/5, Logical Operator211/5
  Logical Operator217/1 -> Logical Operator220/4
  Alignment67/1 -> Logical Operator224/1, Logical Operator216/4, Logical Operator228/4, Logical Operator226/4, Logical Operator211/4
  Alignment61/1 -> Logical Operator219/1, Logical Operator226/1, Logical Operator213/1, Logical Operator212/1, Logical Operator211/1, Logical Operator210/1, Logical Operator209/1
  Logical Operator222/1 -> Logical Operator231/2, Logical Operator228/2, Logical Operator221/2, Logical Operator212/2, Logical Operator211/2, Logical Operator210/2
  Logical Operator226/1 -> Logical Operator208/1
  Logical Operator205/1 -> Alignment65/1
  Logical Operator231/1 -> Logical Operator230/1
  Logical Operator208/1 -> A = B(1b)/1
  Logical Operator220/1 -> (uint) A < B(1b)/1, Enable unsigned (A < B)/2
  Logical Operator230/1 -> Enable unsigned (2) (A > B)/1, (uint) A > B(1b)/1
  Logical Operator/1 -> Logical Operator326/1
  Logical Operator327/1 -> Logical Operator/1
  Logical Operator325/1 -> Logical Operator303/2
  Logical Operator303/1 -> Logical Operator326/2

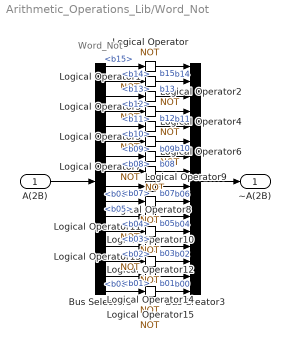
== system Arithmetic_Operations_Lib/Word_Not ==
  note: Word_Not
  A(2B) : Inport
  Bus Creator3 : BusCreator  Inputs=16
  Bus Selector3 : BusSelector  OutputSignals=b15,b14,b13,b12,b11,b10,b09,b08,b07,b06,b05,b04,b03,b02,b01,b00
  Logical Operator{,1..15} (16 alike) : Logic  Operator=NOT  IconShape=distinctive  AllPortsSameDT=off  OutDataTypeStr=boolean
  ~A(2B) : Outport
  wires:
  Bus Creator3/1 -> ~A(2B)/1
  A(2B)/1 -> Bus Selector3/1
  Logical Operator/1 -> Bus Creator3/1  "b15"
  Logical Operator1/1 -> Bus Creator3/2  "b14"
  Logical Operator2/1 -> Bus Creator3/3  "b13"
  Logical Operator7/1 -> Bus Creator3/8  "b08"
  Logical Operator6/1 -> Bus Creator3/7  "b09"
  Logical Operator5/1 -> Bus Creator3/6  "b10"
  Logical Operator3/1 -> Bus Creator3/4  "b12"
  Logical Operator4/1 -> Bus Creator3/5  "b11"
  Bus Selector3/8 -> Logical Operator7/1  "<b08>"
  Bus Selector3/7 -> Logical Operator6/1  "<b09>"
  Bus Selector3/6 -> Logical Operator5/1  "<b10>"
  Bus Selector3/5 -> Logical Operator4/1  "<b11>"
  Bus Selector3/4 -> Logical Operator3/1  "<b12>"
  Bus Selector3/3 -> Logical Operator2/1  "<b13>"
  Bus Selector3/2 -> Logical Operator1/1  "<b14>"
  Bus Selector3/1 -> Logical Operator/1  "<b15>"
  Bus Selector3/16 -> Logical Operator15/1  "<b00>"
  Bus Selector3/15 -> Logical Operator14/1  "<b01>"
  Bus Selector3/14 -> Logical Operator13/1  "<b02>"
  Bus Selector3/13 -> Logical Operator12/1  "<b03>"
  Bus Selector3/12 -> Logical Operator11/1  "<b04>"
  Bus Selector3/11 -> Logical Operator10/1  "<b05>"
  Bus Selector3/10 -> Logical Operator9/1  "<b06>"
  Bus Selector3/9 -> Logical Operator8/1  "<b07>"
  Logical Operator8/1 -> Bus Creator3/9  "b07"
  Logical Operator9/1 -> Bus Creator3/10  "b06"
  Logical Operator10/1 -> Bus Creator3/11  "b05"
  Logical Operator11/1 -> Bus Creator3/12  "b04"
  Logical Operator12/1 -> Bus Creator3/13  "b03"
  Logical Operator13/1 -> Bus Creator3/14  "b02"
  Logical Operator14/1 -> Bus Creator3/15  "b01"
  Logical Operator15/1 -> Bus Creator3/16  "b00"
